simulink model "controle_03"  (R2015a)
settings: Solver=ode45  StartTime=0.0  StopTime=t_run  FixedStep=1e-3  RelTol=1e-6
values from neighbouring files (symbols this model uses):
  G = 1/(s*(s+1))    [sim_01.m]
  t_step = 1    [sim_01.m]
  Ts = 0.01    [pid_custom.m]
settings Model: CovSFcnEnable=off  Creator=angelico  LastModifiedBy=Convidado do LCA
settings DataIOCC: SignalLoggingSaveFormat=ModelDataLogs
settings OptimizationCC: ExpressionDepthLimit=2147483647
settings DebuggingCC: UnderspecifiedInitializationDetection=Classic  MergeDetectMultiDrivingBlocksExec=none  SolverPrmCheckMsg=warning  FcnCallInpInsideContextMsg=UseLocalSettings  StateNameClashWarn=warning
settings GRTTargetCC: CombineOutputUpdateFcns=off  GRTInterface=on

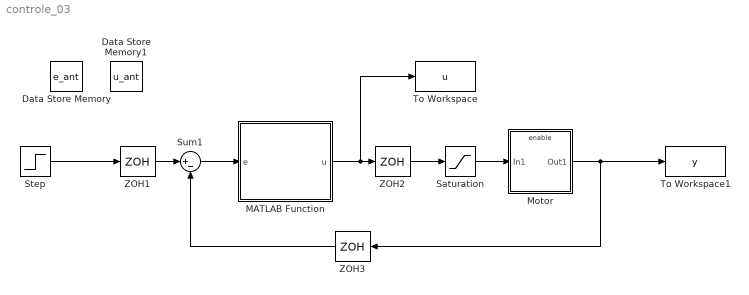
== system controle_03 ==
  Data Store Memory : DataStoreMemory  DataStoreName=e_ant  ReadBeforeWriteMsg=warning  WriteAfterWriteMsg=warning  WriteAfterReadMsg=warning  OutDataTypeStr=double
  Data Store Memory1 : DataStoreMemory  DataStoreName=u_ant  ReadBeforeWriteMsg=warning  WriteAfterWriteMsg=warning  WriteAfterReadMsg=warning  OutDataTypeStr=double
  MATLAB Function : MATLAB Function  TreatAsAtomicUnit=on
  Motor : Subsystem
  Saturation : Saturate  UpperLimit=50  LowerLimit=-50
  Step : Step  Time=t_step  SampleTime=Ts
  Sum1 : Sum  Inputs=|+-  SampleTime=Ts
  To Workspace : ToWorkspace  VariableName=u  SampleTime=-1
  To Workspace1 : ToWorkspace  VariableName=y  SampleTime=-1
  ZOH1 : ZeroOrderHold  SampleTime=Ts
  ZOH2 : ZeroOrderHold  SampleTime=Ts
  ZOH3 : ZeroOrderHold  SampleTime=Ts
  wires:
  Step/1 -> ZOH1/1
  Sum1/1 -> MATLAB Function/1(e)
  MATLAB Function/1(u) -> To Workspace/1, ZOH2/1
  ZOH3/1 -> Sum1/2
  ZOH1/1 -> Sum1/1
  Motor/1(Out1) -> To Workspace1/1, ZOH3/1
  ZOH2/1 -> Saturation/1
  Saturation/1 -> Motor/1(In1)

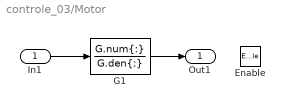
== system controle_03/Motor ==
  In1 : Inport
  Enable : EnablePort
  G1 : TransferFcn  Numerator=G.num{:}  Denominator=G.den{:}
  Out1 : Outport
  wires:
  In1/1 -> G1/1
  G1/1 -> Out1/1

== matlab function controle_03/MATLAB Function ==
  settings: updateMethod=DISCRETE  sampleTime=Ts
  data: u output; e input; param parameter; u_ant data_store_memory; e_ant data_store_memory
function u  = fcn(e,param)

global u_ant; global e_ant;

a = param(1); b = param(2); K = param(3);
u = b*u_ant + K*e - K*a*e_ant;
u_ant = u; e_ant = e;

end
